simulink model "Linear_System_report"  (R2019b)
settings: Solver=FixedStepAuto  StartTime=0.0  StopTime=50  FixedStep=1e-3  RelTol=1e-3
values from neighbouring files (symbols this model uses):
  A = [ 0 1 0 0 ... (first row only)    [parameters.m]
  B = [0 ... (first row only)    [parameters.m]
  C = eye(4)    [parameters.m]
  D = zeros(4,1)    [parameters.m]
  ini_cond = [0 0 pi/3 0]'    [parameters.m]
  K = lqr(A,B,Q,R)    [parameters.m]
  Kt = 0.0833    [parameters.m]
libraries: simulink x1
settings Model: Creator=nikhita  LastModifiedBy=nikhita
settings SFSimCC: CustomCodeUndefinedFunction=UseInterfaceOnly

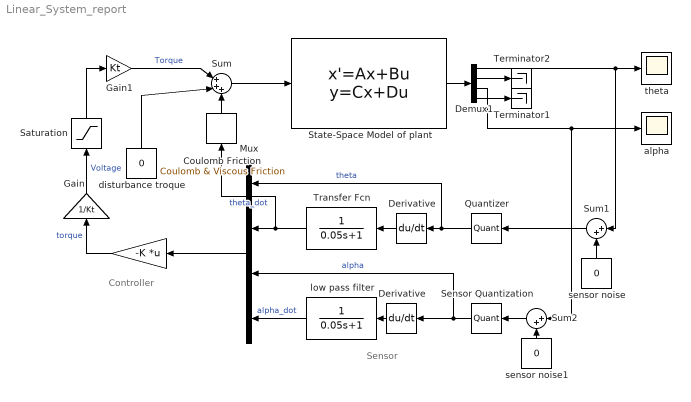
== system Linear_System_report ==
  note: Controller
  note: Sensor
  " " : Gain  Gain=-K  Multiplication=Matrix(K*u)
  " disturbance troque" : Constant  Value=0
  " theta " : Scope
  Coulomb Friction : simulink/Discontinuities/Coulomb & Viscous Friction  offset=[0]  gain=0
      settings: SourceProductName=Simulink
  Demux1 : Demux
  Derivative : Derivative  CoefficientInTFapproximation=0
  "Derivative " : Derivative  CoefficientInTFapproximation=0
  Gain : Gain  Gain=1/Kt
  Gain1 : Gain  Gain=Kt
  Mux : Mux
  Quantizer : Quantizer  QuantizationInterval=0.0018*pi/180
  "Saturation " : Saturate  UpperLimit=3  LowerLimit=-3
  Sensor Quantization : Quantizer  QuantizationInterval=0.0018*pi/180
  State-Space Model of plant : StateSpace  A=A  B=B  C=C  D=D  InitialCondition=ini_cond
  Sum : Sum  Inputs=|+++
  Sum1 : Sum  Inputs=|++
  Sum2 : Sum  Inputs=|++
  Terminator1 : Terminator
  Terminator2 : Terminator
  Transfer Fcn : TransferFcn  Denominator=[0.05 1]
  "alpha " : Scope
  low pass filter : TransferFcn  Denominator=[0.05 1]
  sensor noise : Constant  Value=0
  sensor noise1 : Constant  Value=0
  wires:
  State-Space Model of plant/1 -> Demux1/1
  " "/1 -> Gain/1  "torque"
  Demux1/1 -> " theta "/1, Sum1/1
  Demux1/3 -> Sum2/1, "alpha "/1
  Quantizer/1 -> Derivative/1, Mux/1  "theta"
  Mux/1 -> " "/1
  Derivative/1 -> Transfer Fcn/1
  Sensor Quantization/1 -> Mux/3, "Derivative "/1  "alpha"
  "Derivative "/1 -> low pass filter/1
  Transfer Fcn/1 -> Coulomb Friction/1, Mux/2  "theta_dot"
  low pass filter/1 -> Mux/4  "alpha_dot"
  Demux1/2 -> Terminator2/1
  Demux1/4 -> Terminator1/1
  "Saturation "/1 -> Gain1/1
  Gain/1 -> "Saturation "/1  "Voltage"
  Gain1/1 -> Sum/1  "Torque"
  Sum/1 -> State-Space Model of plant/1
  " disturbance troque"/1 -> Sum/2
  sensor noise/1 -> Sum1/2
  Sum1/1 -> Quantizer/1
  sensor noise1/1 -> Sum2/2
  Sum2/1 -> Sensor Quantization/1
  Coulomb Friction/1 -> Sum/3
